simulink model "TrajectoryControl"  (R2018b)
settings: Solver=ode3  StartTime=0.0  StopTime=100.0  FixedStep=Ts  RelTol=1e-3
values from neighbouring files (symbols this model uses):
  th_0 = 0    [Ejercicio2.m]
  Ts = 100e-3    (= 0.1)    [Ejercicio1.m]    (also in Ejercicio2.m)
  x_0 = 0    [Ejercicio2.m]
  y_0 = 0    [Ejercicio2.m]
undefined symbols (not defined in the file or in its folder): DiscIntNeverNeededParam, sigbuilder_block
libraries: simulink x1, fuzblock x1
settings Model: EnablePacing=on  PacingRate=10  Creator=Edu  LastModifiedBy=Edu

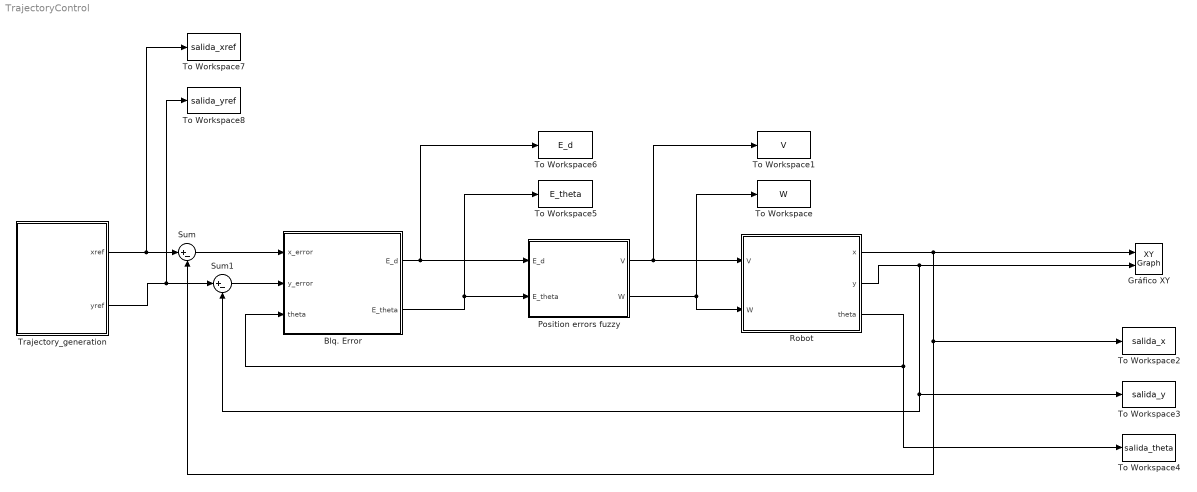
== system TrajectoryControl ==
  Blq. Error : Subsystem
  Gráfico XY : simulink/Sinks/XY Graph  xmin=-5  xmax=5  ymin=-5  ymax=5  st=-1
  Position errors fuzzy : Subsystem
  Robot : Subsystem
  Sum : Sum  Inputs=|+-
  Sum1 : Sum  Inputs=|+-
  To Workspace : ToWorkspace  VariableName=W  SaveFormat=Structure With Time  SampleTime=-1
  To Workspace1 : ToWorkspace  VariableName=V  SaveFormat=Structure With Time  SampleTime=-1
  To Workspace2 : ToWorkspace  VariableName=salida_x  SaveFormat=Structure With Time  SampleTime=-1
  To Workspace3 : ToWorkspace  VariableName=salida_y  SaveFormat=Structure With Time  SampleTime=-1
  To Workspace4 : ToWorkspace  VariableName=salida_theta  SaveFormat=Structure With Time  SampleTime=-1
  To Workspace5 : ToWorkspace  VariableName=E_theta  SaveFormat=Structure With Time  SampleTime=-1
  To Workspace6 : ToWorkspace  VariableName=E_d  SaveFormat=Structure With Time  SampleTime=-1
  To Workspace7 : ToWorkspace  VariableName=salida_xref  SaveFormat=Structure With Time  SampleTime=-1
  To Workspace8 : ToWorkspace  VariableName=salida_yref  SaveFormat=Structure With Time  SampleTime=-1
  Trajectory_generation : Subsystem
  wires:
  Robot/1(x) -> Gráfico XY/1, To Workspace2/1, Sum/2
  Robot/2(y) -> Gráfico XY/2, To Workspace3/1, Sum1/2
  Robot/3(theta) -> Blq. Error/3(theta), To Workspace4/1
  Blq. Error/2(E_theta) -> Position errors fuzzy/2(E_theta), To Workspace5/1
  Blq. Error/1(E_d) -> Position errors fuzzy/1("E_d "), To Workspace6/1
  Position errors fuzzy/1(V) -> To Workspace1/1, Robot/1(V)
  Position errors fuzzy/2("W ") -> Robot/2(W), To Workspace/1
  Sum/1 -> Blq. Error/1(x_error)
  Sum1/1 -> Blq. Error/2(y_error)
  Trajectory_generation/1(xref) -> To Workspace7/1, Sum/1
  Trajectory_generation/2(yref) -> To Workspace8/1, Sum1/1

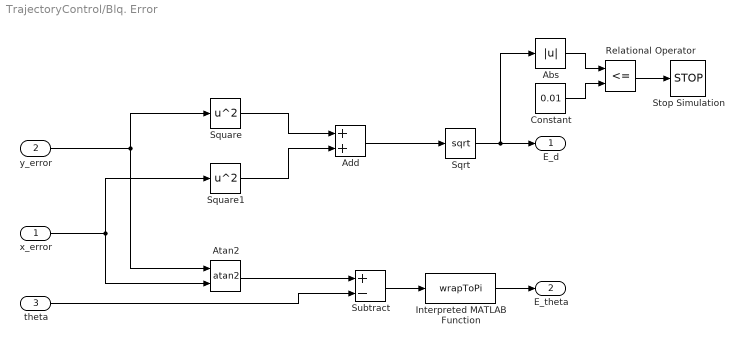
== system TrajectoryControl/Blq. Error ==
  x_error : Inport
  y_error : Inport  Port=2
  theta : Inport  Port=3
  Abs : Abs
  Add : Sum
  Atan2 : Trigonometry  Operator=atan2
  Constant : Constant  Value=0.01
  Interpreted MATLAB Function : MATLABFcn  MATLABFcn=wrapToPi
  Relational Operator : RelationalOperator  Operator=<=  OutDataTypeStr=boolean  RndMeth=Simplest
  Sqrt : Sqrt  SaturateOnIntegerOverflow=on
  Square : Math  Operator=square  SaturateOnIntegerOverflow=on
  Square1 : Math  Operator=square  SaturateOnIntegerOverflow=on
  Stop Simulation : Stop
  Subtract : Sum  Inputs=+-  OutMin=[-3.14]  OutMax=[3.14]
  E_d : Outport
  E_theta : Outport  Port=2  OutMin=[-pi]  OutMax=[pi]
  wires:
  y_error/1 -> Atan2/1, Square/1
  x_error/1 -> Atan2/2, Square1/1
  Square/1 -> Add/1
  Square1/1 -> Add/2
  Add/1 -> Sqrt/1
  Sqrt/1 -> Abs/1, E_d/1
  Atan2/1 -> Subtract/1
  theta/1 -> Subtract/2
  Abs/1 -> Relational Operator/1
  Constant/1 -> Relational Operator/2
  Relational Operator/1 -> Stop Simulation/1
  Interpreted MATLAB Function/1 -> E_theta/1
  Subtract/1 -> Interpreted MATLAB Function/1

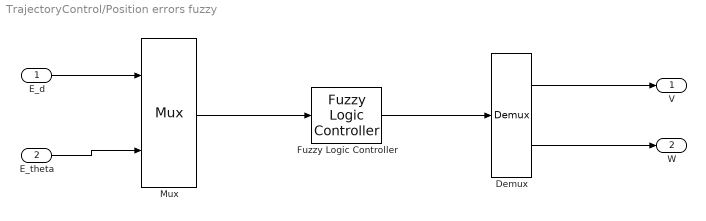
== system TrajectoryControl/Position errors fuzzy ==
  "E_d " : Inport
  E_theta : Inport  Port=2
  Demux : Demux  Outputs=2
  Fuzzy Logic Controller : fuzblock/Fuzzy Logic  Controller  FIS='ControlBorroso.fis'  OutputSampleNumber=101  DataType=double  FuzzifiedInputs=off  RuleFiringStrengths=off  RuleOutputs=off  AggregatedOutputs=off  SimulateUsing=Interpreted execution  OutOfRangeInputValueMessage=warning  NoRuleFiredMessage=warning  EmptyOutputFuzzySetMessage=warning
  Mux : Mux  Inputs=2
  V : Outport
  "W " : Outport  Port=2
  wires:
  Mux/1 -> Fuzzy Logic Controller/1
  "E_d "/1 -> Mux/1
  Demux/1 -> V/1
  Demux/2 -> "W "/1
  E_theta/1 -> Mux/2
  Fuzzy Logic Controller/1 -> Demux/1

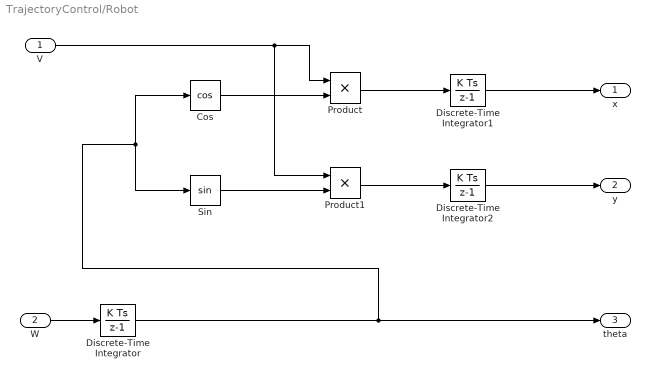
== system TrajectoryControl/Robot ==
  V : Inport
  W : Inport  Port=2
  Cos : Trigonometry  Operator=cos
  Discrete-Time Integrator : DiscreteIntegrator  SampleTime=-1  ICPrevOutput=DiscIntNeverNeededParam  ICPrevScaledInput=DiscIntNeverNeededParam
  Discrete-Time Integrator1 : DiscreteIntegrator  InitialCondition=-1  SampleTime=-1  ICPrevOutput=DiscIntNeverNeededParam  ICPrevScaledInput=DiscIntNeverNeededParam
  Discrete-Time Integrator2 : DiscreteIntegrator  InitialCondition=-1  SampleTime=-1  ICPrevOutput=DiscIntNeverNeededParam  ICPrevScaledInput=DiscIntNeverNeededParam
  Product : Product
  Product1 : Product
  Sin : Trigonometry
  x : Outport
  y : Outport  Port=2
  theta : Outport  Port=3
  wires:
  Sin/1 -> Product1/2
  Product1/1 -> Discrete-Time Integrator2/1
  Product/1 -> Discrete-Time Integrator1/1
  Discrete-Time Integrator2/1 -> y/1
  V/1 -> Product1/1, Product/1
  Discrete-Time Integrator1/1 -> x/1
  Discrete-Time Integrator/1 -> theta/1, Sin/1, Cos/1
  W/1 -> Discrete-Time Integrator/1
  Cos/1 -> Product/2

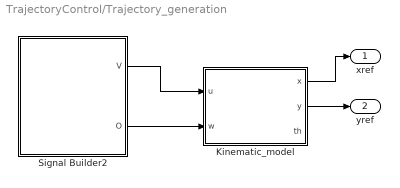
== system TrajectoryControl/Trajectory_generation ==
  Kinematic_model : Subsystem
  Signal Builder2 : Subsystem  Tag=STV Subsys  LoadFcn=sigbuilder_block('load');  StartFcn=sigbuilder_block('start');  StopFcn=sigbuilder_block('stop');  ClipboardFcn=sigbuilder_block('clipboard');  mask(Sigbuilder block){tuvar=[0:10]}
      mask help: Sigbuilder GUI
      mask init:
      | if ~strcmp(get_param(bdroot(gcbh),'SimulationStatus'),'stopped') tuvar = sigbuilder_block('maskInit'); end
      settings: CopyFcn=sigbuilder_block('copy');  DeleteFcn=sigbuilder_block('delete');  ModelCloseFcn=sigbuilder_block('modelClose');  PreSaveFcn=sigbuilder_block('preSave');  PauseFcn=sigbuilder_block('pause')  ContinueFcn=sigbuilder_block('continue')  NameChangeFcn=sigbuilder_block('namechange');  OpenFcn=sigbuilder_block('open',[60 45 534.4 467.25 ]);  CloseFcn=sigbuilder_block('close');
      mask Display: plot(0, 0, 100, 100,[2, 2, 32, 32, 2], [68, 8, 8, 68, 68],[32, 2], [38, 38], [32, 19, 2],[53, 60, 44], [32, 17, 17, 2],[16, 16, 31, 31]);txt = getActiveGroup(gcbh);text(2, 100, txt,'verticalAlignment', 'top');
  xref : Outport
  yref : Outport  Port=2
  wires:
  Kinematic_model/2(y) -> yref/1
  Kinematic_model/1(x) -> xref/1
  Signal Builder2/2(O) -> Kinematic_model/2(w)
  Signal Builder2/1(V) -> Kinematic_model/1(u)

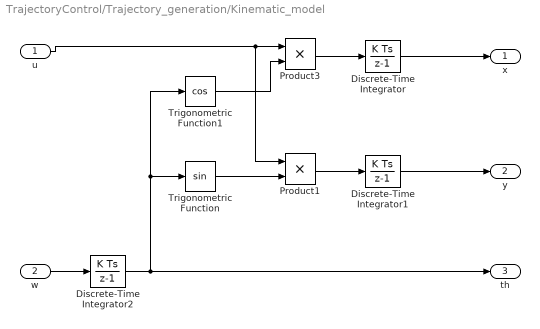
== system TrajectoryControl/Trajectory_generation/Kinematic_model ==
  u : Inport
  w : Inport  Port=2
  Discrete-Time Integrator : DiscreteIntegrator  InitialCondition=x_0  SampleTime=Ts  ICPrevOutput=DiscIntNeverNeededParam  ICPrevScaledInput=DiscIntNeverNeededParam
  Discrete-Time Integrator1 : DiscreteIntegrator  InitialCondition=y_0  SampleTime=Ts  ICPrevOutput=DiscIntNeverNeededParam  ICPrevScaledInput=DiscIntNeverNeededParam
  Discrete-Time Integrator2 : DiscreteIntegrator  InitialCondition=th_0  SampleTime=Ts  ICPrevOutput=DiscIntNeverNeededParam  ICPrevScaledInput=DiscIntNeverNeededParam
  Product1 : Product
  Product3 : Product
  Trigonometric Function : Trigonometry
  Trigonometric Function1 : Trigonometry  Operator=cos
  x : Outport
  y : Outport  Port=2
  th : Outport  Port=3
  wires:
  Discrete-Time Integrator/1 -> x/1
  Discrete-Time Integrator1/1 -> y/1
  Trigonometric Function1/1 -> Product3/2
  u/1 -> Product3/1, Product1/1
  Trigonometric Function/1 -> Product1/2
  w/1 -> Discrete-Time Integrator2/1
  Product3/1 -> Discrete-Time Integrator/1
  Product1/1 -> Discrete-Time Integrator1/1
  Discrete-Time Integrator2/1 -> th/1, Trigonometric Function/1, Trigonometric Function1/1

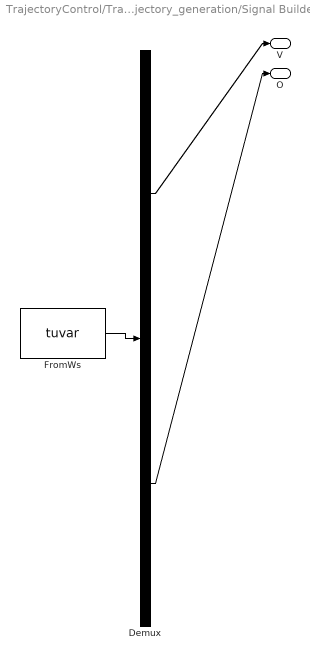
== system TrajectoryControl/Trajectory_generation/Signal Builder2 ==
  Demux : Demux  Tag=STV Demux  Outputs=2
  FromWs : FromWorkspace  Tag=STV FromWs  VariableName=tuvar  SampleTime=0
      SigBuilderData=|
      | common.afterFinalStr = 'Extrapolate'
      | common.sampleTime = '0'
      | dataSet.timeRange = [0 115]
      | dataSet.name = 'Group 1'
      | sbobj.Groups.Name = 'Group 1'
      | sbobj.Groups.Signals(1).Name = 'V'
      | sbobj.Groups.Signals(1).XData = [0 87 87 115]
      | sbobj.Groups.Signals(1).YData = [0.25 0.25 0 0]
      | sbobj.Groups.Signals(2).Name = 'O'
      | sbobj.Groups.Signals(2).XData = [0 12 12 30.849 30.849 55.981 55.981 74.83 74.83 99.962 115]
      | sbobj.Groups.Signals(2).YData = [0 0 0.25 0.25 -0.25 -0.25 0.25 0.25 0 0 0]
      | sbobj.Groups.TimeRange = [0 115]
  V : Outport  Tag=STV Outport
  O : Outport  Tag=STV Outport  Port=2
  wires:
  Demux/2 -> O/1
  Demux/1 -> V/1
  FromWs/1 -> Demux/1
